simulink library "Power_Shaft2_Electric_L2_R2"  (R2022b)
settings: Solver=VariableStepAuto  StartTime=0.0  StopTime=10.0  RelTol=1e-3
values from neighbouring files (symbols this model uses):
  VDatabase = evalin('base','VDatabase')    [sm_car_controlparam_Electric_A1_A2_default.m]
undefined symbols (not defined in the file or in its folder): ShaftL2, ShaftR2
libraries: Power_Components x3, fl_lib x2, sm_lib x1, Cooling_Motor2_L2R2 x1
Description:
  | Component of Simscape Vehicle Templates Library
  | 
  | Copyright 2018-2024 The MathWorks, Inc.
settings Model: Creator=smiller  LastModifiedBy=smiller
settings SolverCC: AlgebraicLoopSolver=TrustRegion
settings DataIOCC: ReturnWorkspaceOutputs=off
settings DebuggingCC: UnconnectedInputMsg=warning  UnconnectedOutputMsg=warning  UnconnectedLineMsg=warning  SFMachineParentedDataDiag=warning  ArithmeticOperatorsInVariantConditions=warning
settings ModelReferenceCC: EnableRefExpFcnMdlSchedulingChecks=on
settings SFSimCC: CustomCodeUndefinedFunction=UseInterfaceOnly

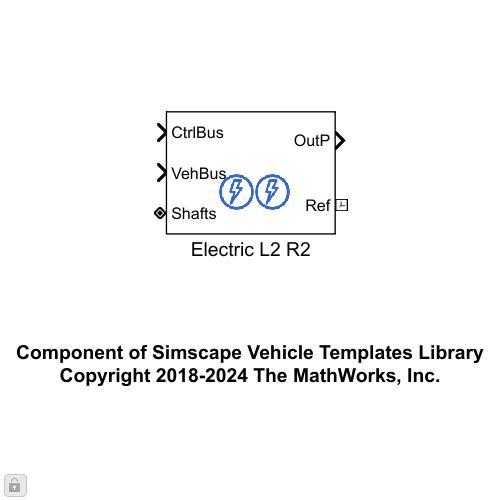
[thumbnail: Simulink's stored preview of the top-level diagram]
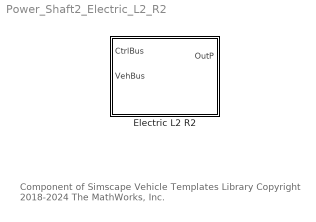
== system Power_Shaft2_Electric_L2_R2 ==
  note: Component of Simscape Vehicle Templates Library
      | Copyright 2018-2024 The MathWorks, Inc.
  Electric L2 R2 : Subsystem  mask(Electric Propulsion with Two Motors (RWD)){Power=VDatabase.Power.Electric2Motor_L2_R2_default}
      mask prompts: Power "Power 2 Motor (structure)"
      mask help: Two electric motors with optional cooling system. Physical connections for the two motor shafts are in bus Shafts and connect to the left and right rear wheels.
      mask Display: image('sm_car_vehicle_power_e2motor_L2R2_IMAGE.png');

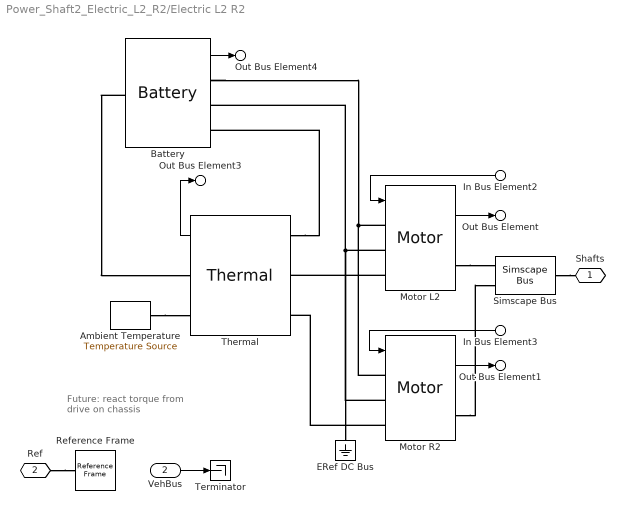
== system Power_Shaft2_Electric_L2_R2/Electric L2 R2 ==
  note: Future:
      | react torque
      | from drive
      | on chassis
  In Bus Element2 : Inport  PortName=CtrlBus  Element=MMotorL2Demand
  In Bus Element3 : Inport  PortName=CtrlBus  Element=MMotorR2Demand
  VehBus : Inport  Port=2
  Ambient Temperature : fl_lib/Thermal/Thermal Sources/Temperature Source  temperature=Power.TAmbient.Value K
  Battery : Power_Components/Battery  SystemSampleTime=-1  VariantActivationTime=update diagram  Latency=0  AutoFrameSizeCalculation=off
  ERef DC Bus : fl_lib/Electrical/Electrical Elements/Electrical Reference
  Motor L2 : Power_Components/Motor  Motor=Power.MotorL2
  Motor R2 : Power_Components/Motor  Motor=Power.MotorL2
  Reference Frame : sm_lib/Frames and Transforms/Reference Frame
  Simscape Bus : SimscapeBus  HierarchyStrings=ShaftL2;ShaftR2
  Terminator : Terminator
  Thermal : Cooling_Motor2_L2R2/Thermal  VariantControl=Variant1  LabelModeActiveChoice=Liquid_Loop1  VariantLabel=Power.Cooling.class.Value
      settings: AttributesFormatString=%<ActiveVariant>
  Shafts : PMIOPort  Side=Left
  Ref : PMIOPort  Port=2  Side=Right
  Out Bus Element : Outport  VectorParamsAs1DForOutWhenUnconnected=off  PortName=OutP  Element=MotorL2
  Out Bus Element1 : Outport  VectorParamsAs1DForOutWhenUnconnected=off  PortName=OutP  Element=MotorR2
  Out Bus Element3 : Outport  VectorParamsAs1DForOutWhenUnconnected=off  PortName=OutP  Element=Thermal
  Out Bus Element4 : Outport  VectorParamsAs1DForOutWhenUnconnected=off  PortName=OutP  Element=Battery
  wires:
  In Bus Element2/1 -> Motor L2/1
  Motor L2/1 -> Out Bus Element/1
  Motor R2/1 -> Out Bus Element1/1
  In Bus Element3/1 -> Motor R2/1
  Thermal/1 -> Out Bus Element3/1
  VehBus/1 -> Terminator/1
  Battery/1 -> Out Bus Element4/1
  connections:
  Motor R2/RConn1 -- Simscape Bus/LConn2
  Motor L2/LConn2 -- Motor R2/LConn2 -- ERef DC Bus/LConn1 -- Battery/RConn2
  Motor L2/LConn1 -- Battery/RConn1 -- Motor R2/LConn1
  Motor L2/RConn1 -- Simscape Bus/LConn1
  Simscape Bus/RConn1 -- Shafts/RConn1
  Ref/RConn1 -- Reference Frame/RConn1
  Motor L2/LConn3 -- Thermal/LConn2
  Motor R2/LConn3 -- Thermal/LConn3
  Ambient Temperature/LConn1 -- Thermal/RConn2
  Thermal/LConn1 -- Battery/RConn3
  Battery/LConn1 -- Thermal/RConn1
